simulink model "One_Three_Phase_Transformer"  (R2024a)
settings: Solver=ode23tb  StartTime=0.0  StopTime=0.2  MaxStep=1e-4  RelTol=1e-3
libraries: spsRMSLib x4, spsACVoltageSourceLib x3, spsThreePhaseVIMeasurementLib x2, spsGroundLib x1, spsThreePhaseSeriesRLCLoadLib x1, spsThreePhaseTransformerTwoWindingsLib x1, sps_lib x1
settings Model: Creator=91889  LastModifiedBy=91889

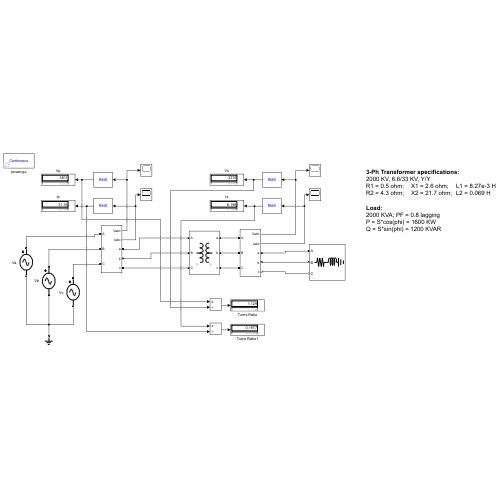
[thumbnail: Simulink's stored preview of the top-level diagram]
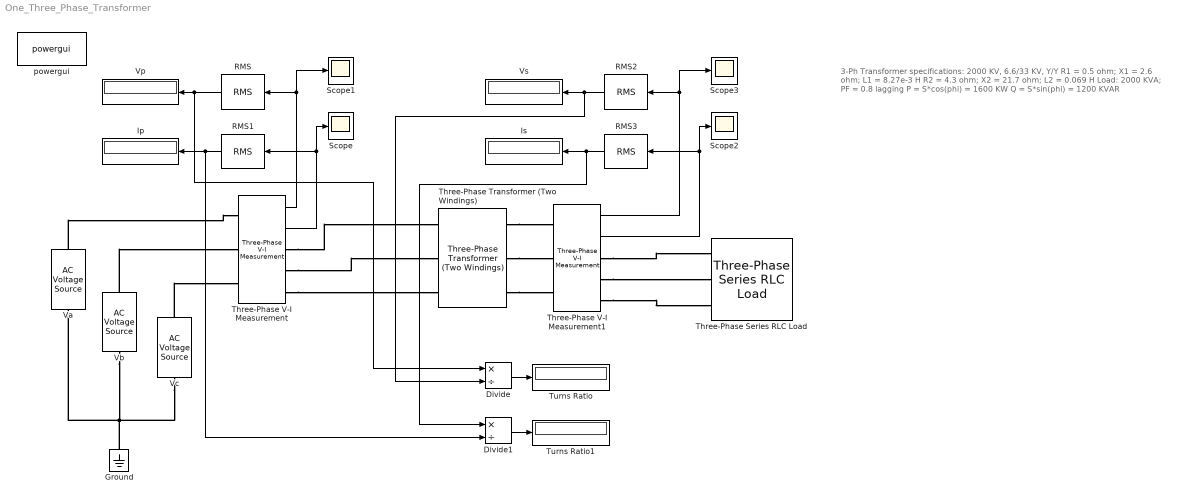
== system One_Three_Phase_Transformer ==
  note: 3-Ph Transformer specifications:
      | 2000 KV, 6.6/33 KV, Y/Y
      | R1 = 0.5 ohm; X1 = 2.6 ohm; L1 = 8.27e-3 H
      | R2 = 4.3 ohm; X2 = 21.7 ohm; L2 = 0.069 H
      |
      | Load:
      | 2000 KVA; PF = 0.8 lagging
      | P = S*cos(phi) = 1600 KW
      | Q = S*sin(phi) = 1200 KVAR
  Divide : Product  Inputs=*/
  Divide1 : Product  Inputs=*/
  Ground : spsGroundLib/Ground  LConnTagsString=a
  Ip : Display
  Is : Display
  RMS{,1..3} (4 alike) : spsRMSLib/RMS  TrueRMS=on  Freq=50  RMSInit=0  Ts=0
  Scope{,1..3} (4 alike) : Scope
  Three-Phase Series RLC Load : spsThreePhaseSeriesRLCLoadLib/Three-Phase Series RLC Load  LConnTagsString=A|B|C  Configuration=Y (grounded)  NominalVoltage=33e3  Vabc=[1e3 1e3 1e3]  Vabcp=[1e3 1e3 1e3]  NominalFrequency=50  UnbalancedPower=off  ActivePower=1600e3  InductivePower=1200e3  CapacitivePower=0  Pabc=[10e3 9e3 11e3]  QLabc=[100 90 110]  QCabc=[100 90 110]  Pabcp=[10e3 9e3 11e3]  QLabcp=[100 90 110]  QCabcp=[100 90 110]  Measurements=None  LoadType=constant Z
  Three-Phase Transformer (Two Windings) : spsThreePhaseTransformerTwoWindingsLib/Three-Phase Transformer (Two Windings)  Winding1Connection=Y  Winding2Connection=Y  CoreType=Three single-phase transformers  SetSaturation=off  Hysteresis=off  DataFile='hysteresis'  SetInitialFlux=off  Measurements=None  UNITS=pu  NominalPower=[ 2000e3 , 50 ]  Winding1=[6.6e3 , 0.5 , 8.27e-3 ]  Winding2=[ 33e3 , 4.3 , 0.069 ]  Rm=500  Lm=500  L0=0.5  Saturation=[ 0,0 ; 0.0024,1.2 ; 1.0,1.52 ]  InitialFluxes=[ 0.8 , -0.8 , 0.7 ]  BreakLoop=off  DiscreteSolver=Trapezoidal iterative  DataType=off  TransfoNumber=1
  Three-Phase V-I Measurement : spsThreePhaseVIMeasurementLib/Three-Phase V-I Measurement  VoltageMeasurement=phase-to-ground  SetLabelV=off  LabelV=Vabc  Vpu=off  VpuLL=off  CurrentMeasurement=yes  SetLabelI=off  LabelI=Iabc  Ipu=off  Pbase=100e6  Vbase=500e3  OutputType=Complex  PhasorSimulation=off  PSBequivalent=0
  Three-Phase V-I Measurement1 : spsThreePhaseVIMeasurementLib/Three-Phase V-I Measurement  VoltageMeasurement=phase-to-ground  SetLabelV=off  LabelV=Vabc  Vpu=off  VpuLL=off  CurrentMeasurement=yes  SetLabelI=off  LabelI=Iabc  Ipu=off  Pbase=100e6  Vbase=500e3  OutputType=Complex  PhasorSimulation=off  PSBequivalent=0
  Turns Ratio : Display
  Turns Ratio1 : Display
  Va : spsACVoltageSourceLib/AC Voltage Source  Amplitude=6.6e3*sqrt(2)/sqrt(3)  Phase=0  Frequency=50  SampleTime=0  Measurements=None  BusType=swing  Pref=10e3  Qref=0  Qmin=-inf  Qmax=+inf
  Vb : spsACVoltageSourceLib/AC Voltage Source  Amplitude=6.6e3*sqrt(2)/sqrt(3)  Phase=-120  Frequency=50  SampleTime=0  Measurements=None  BusType=swing  Pref=10e3  Qref=0  Qmin=-inf  Qmax=+inf
  Vc : spsACVoltageSourceLib/AC Voltage Source  Amplitude=6.6e3*sqrt(2)/sqrt(3)  Phase=120  Frequency=50  SampleTime=0  Measurements=None  BusType=swing  Pref=10e3  Qref=0  Qmin=-inf  Qmax=+inf
  Vp : Display
  Vs : Display
  powergui : sps_lib/powergui  Priority=1  SimulationMode=Continuous  SampleTime=50e-6  frequency=60  Iterations=50  frequencyindice=50  Pbase=100e6  ErrMax=1e-4  UnitsV=kV  UnitsW=MW  buscounter=0  FunctionMessages=off  echomessages=off  EnableUseOfTLC=off  CurrentSourceSwitches=off  DisableSnubberDevices=off  DisableRonSwitches=off  DisableVfSwitches=off  DisplayEquations=off  AutomaticDiscreteSolvers=off  SolverType=Tustin/Backward Euler (TBE)  Interpol=off  ExternalGateDelay=off  methode=off  Ts=100  x0status=blocks  SPID=on  SwTol=0  HookPort=off  NonlinearTolerance=1e-4  nMaxIteration=100  ContinueOnMaxIteration=off  RestoreLinks=warning  ResistiveCurrentMeasurement=off  Frange=[0:2:500]  Ylog=off  Xlog=on  ShowGrid=off  save=off  variable=ZData  structure=0  ZoomFFT=off  StartTime=0.0  cycles=1  DisplayStyle=1  fundamental=60  FreqAxis=off  MaxFrequency=1000  frequencyindicesteady=1  RmsSteady=1  display=off
  wires:
  Three-Phase V-I Measurement/2 -> RMS1/1, Scope/1
  Three-Phase V-I Measurement/1 -> RMS/1, Scope1/1
  RMS/1 -> Divide/1, Vp/1
  RMS1/1 -> Ip/1, Divide1/2
  RMS3/1 -> Divide1/1, Is/1
  Three-Phase V-I Measurement1/1 -> Scope3/1, RMS2/1
  Three-Phase V-I Measurement1/2 -> Scope2/1, RMS3/1
  RMS2/1 -> Vs/1, Divide/2
  Divide/1 -> Turns Ratio/1
  Divide1/1 -> Turns Ratio1/1
  connections:
  Vc/LConn1 -- Ground/LConn1 -- Vb/LConn1 -- Va/LConn1
  Va/RConn1 -- Three-Phase V-I Measurement/LConn1
  Vb/RConn1 -- Three-Phase V-I Measurement/LConn2
  Vc/RConn1 -- Three-Phase V-I Measurement/LConn3
  Three-Phase V-I Measurement/RConn1 -- Three-Phase Transformer (Two Windings)/LConn1
  Three-Phase V-I Measurement/RConn2 -- Three-Phase Transformer (Two Windings)/LConn2
  Three-Phase V-I Measurement/RConn3 -- Three-Phase Transformer (Two Windings)/LConn3
  Three-Phase Transformer (Two Windings)/RConn1 -- Three-Phase V-I Measurement1/LConn1
  Three-Phase Transformer (Two Windings)/RConn2 -- Three-Phase V-I Measurement1/LConn2
  Three-Phase Transformer (Two Windings)/RConn3 -- Three-Phase V-I Measurement1/LConn3
  Three-Phase V-I Measurement1/RConn1 -- Three-Phase Series RLC Load/LConn1
  Three-Phase V-I Measurement1/RConn2 -- Three-Phase Series RLC Load/LConn2
  Three-Phase V-I Measurement1/RConn3 -- Three-Phase Series RLC Load/LConn3
